simulink model "cordic_opt_fixpt16"  (R2021b)
settings: Solver=VariableStepAuto  StartTime=0.0  StopTime=116  RelTol=1e-3
undefined symbols (not defined in the file): S, vsva2197, xcvc1902
libraries: hdlBasic x7, hdlDSPIP x1, vmcUtilities x1
settings Model: Creator=shu_abe  LastModifiedBy=shu_abe

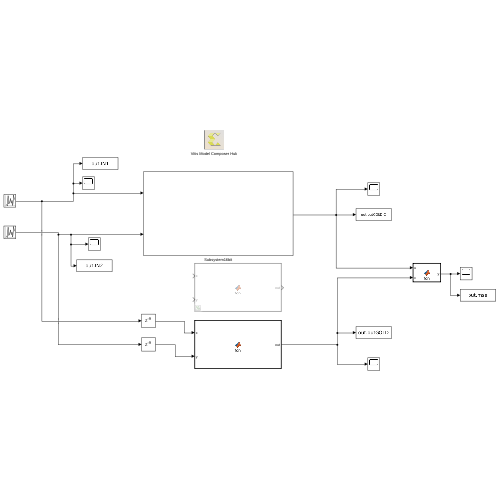
[thumbnail: Simulink's stored preview of the top-level diagram]
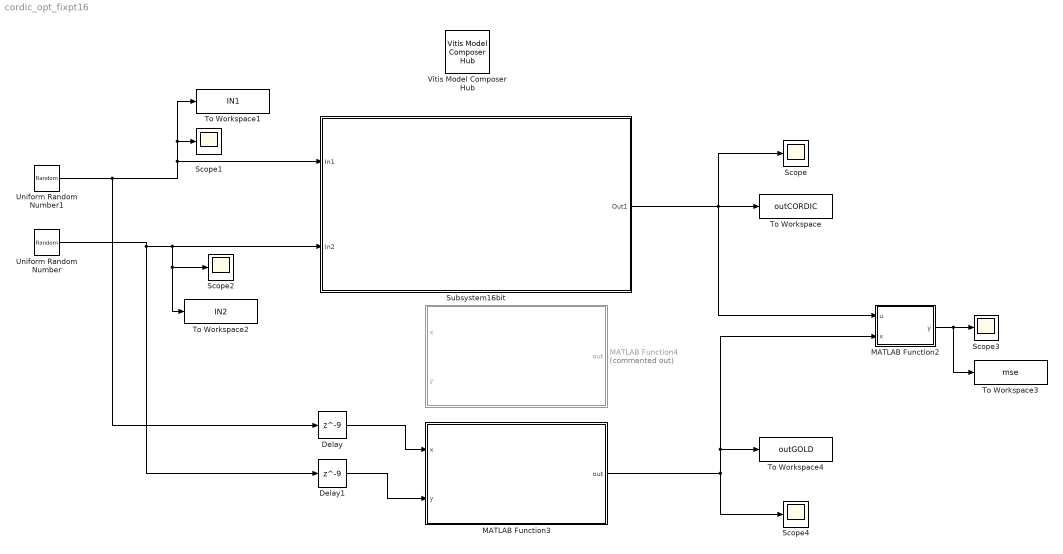
== system cordic_opt_fixpt16 ==
  Delay : Delay  DelayLength=9
  Delay1 : Delay  DelayLength=9
  MATLAB Function2 : MATLAB Function  TreatAsAtomicUnit=on
  MATLAB Function3 : MATLAB Function  TreatAsAtomicUnit=on
  MATLAB Function4 : MATLAB Function  Commented=on  TreatAsAtomicUnit=on
  Scope{,1..4} (5 alike) : Scope
  Subsystem16bit : Subsystem
      mask Display: %%%%
  To Workspace : ToWorkspace  VariableName=outCORDIC  SaveFormat=Structure With Time  SampleTime=-1
  To Workspace1 : ToWorkspace  VariableName=IN1  SaveFormat=Structure With Time  SampleTime=-1
  To Workspace2 : ToWorkspace  VariableName=IN2  SaveFormat=Structure With Time  SampleTime=-1
  To Workspace3 : ToWorkspace  VariableName=mse  SaveFormat=Structure With Time  SampleTime=-1
  To Workspace4 : ToWorkspace  VariableName=outGOLD  SaveFormat=Structure With Time  SampleTime=-1
  Uniform Random Number : UniformRandomNumber  Minimum=-0.7  Maximum=0.7  SampleTime=1
  Uniform Random Number1 : UniformRandomNumber  Minimum=-0.7  Maximum=0.7  Seed=1  SampleTime=1
  Vitis Model Composer Hub : vmcUtilities/Vitis Model Composer Hub  Tag=genX  CodeGeneration=off  SubsystemName=<enter or select subsystem name>  TargetDirectory=./code  ExportType=HLS C++ code  IpVendor=xilinx.com  IpLibrary=hls  IpVersion=1.0  IpHWLanguage=Verilog  AieCompilerOptions={}  CreateTestbench=off  TestbenchStackSize=10  RunAieSim=off  AieSimTimeout=50000  RunAieSimProfiling=off  LaunchVitisAnalyzer=off  PlotOutput=off  RunX86Sim=off  X86SimTimeout=10  GenHwImage=off  PlatformType=Not Specified  HwSystemType=Baremetal  HwValidationTarget=hw  ProjDevice=Alveo U250 Data Center Accelerator Card (xcu250-figd2104-2L-e)  ProjDevicePart=xcvc1902-vsva2197-2MP-e-S  SamplePeriod=-1  ClockFrequency=200  DataPathParallelism=1  xilinxfamily=virtexuplus  part=xcu250  speed=-2L-e  package=figd2104  directory=./cordic_optsim16  testbench=on  incr_netlist=off  synthesis_tool=Vivado  clock_wrapper=Clock Enables  dbl_ovrd=According to Block Masks  dcm_input_clock_period=10  sysclk_period=50  simulink_period=1  eval_field=0
  wires:
  Uniform Random Number/1 -> Subsystem16bit/2(In2), To Workspace2/1, Scope2/1, Delay1/1
  Uniform Random Number1/1 -> Subsystem16bit/1(In1), To Workspace1/1, Scope1/1, Delay/1
  Delay1/1 -> MATLAB Function3/2(y)
  Delay/1 -> MATLAB Function3/1(x)
  MATLAB Function3/1(out) -> Scope4/1, To Workspace4/1, MATLAB Function2/2(x)
  Subsystem16bit/1(Out1) -> Scope/1, MATLAB Function2/1(u), To Workspace/1
  MATLAB Function2/1(y) -> To Workspace3/1, Scope3/1

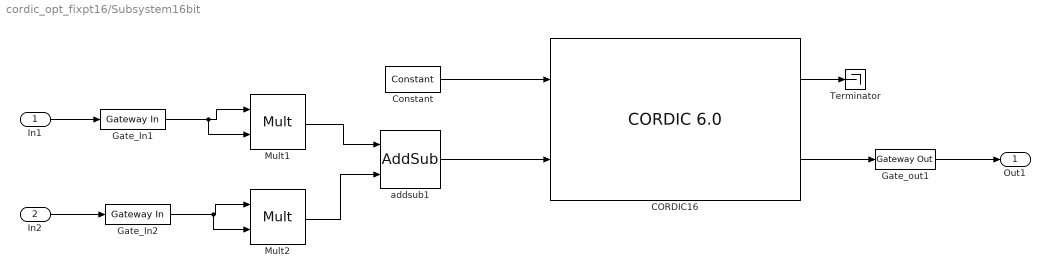
== system cordic_opt_fixpt16/Subsystem16bit ==
  In1 : Inport
  In2 : Inport  Port=2
  CORDIC16 : hdlDSPIP/CORDIC 6.0   functional_selection=Square_Root  architectural_configuration=Parallel  pipelining_mode=Optimal  data_format=UnsignedFraction  phase_format=Radians  input_width=16  output_width=16  round_mode=Round_Pos_Neg_Inf  iterations=0  precision=0  compensation_scaling=No_Scale_Compensation  coarse_rotation=off  aclken=off  aresetn=off  out_tready=off  cartesian_has_tuser=off  cartesian_has_tlast=off  cartesian_tuser_width=1  phase_has_tuser=off  phase_has_tlast=off  phase_tuser_width=1  out_tlast_behv=Null  flow_control=NonBlocking  optimize_goal=Resources  trim_axipin_name=on  simulation_type=hybrid_sim  simulation_model=sysgen:cordic_v6_0  data_path_portlist={'s_axis_cartesian_tdata_imag', 's_axis_cartesian_tdata_real', 's_axis_phase_tdata_phase', 'm_axis_dout_tdata_imag', 'm_axis_dout_tdata_real', 'm_axis_dout_tdata_phase','m_axis_dout_tdata'}  ip_name=CORDIC  ip_version=6.0  dsptool_ready=true  ipcore_usecache=true  ipcore_useipmodelcache=true  wrapper_available=true  port_translation_map={ 'aclken' => 'en', 'aresetn' => 'rst' }  XmcBlockStatus=1  maskContainerNames=group15  block_type=cordic_v6_0  block_config=sysgen:rodinimport_config  block_width=800
  Constant : hdlBasic/Constant  const=1  gui_display_data_type=Boolean  arith_type=Boolean  n_bits=16  bin_pt=14  preci_type=Single  exp_width=8  frac_width=24  explicit_period=on  period=1  XmcBlockStatus=1  maskContainerNames=tabcontainer1  block_type=constant  block_config=sysgen:Constant_config
  Gate_In1 : hdlBasic/Gateway In  gui_display_data_type=Fixed-point  arith_type=Signed (2's comp)  n_bits=16  bin_pt=14  preci_type=Single  exp_width=8  frac_width=24  rows=1  columns=1  quantization="Round  (unbiased: +/- Inf)"  overflow=Saturate  period=1  UseAsADC=off  ADCChannel='1'  interface=None  automatic_assignment=on  address_offset=hex2dec('00')  intf_name=''  intf_description=''  default_value=0  timing_constraint=None  locs_specified=off  LOCs={}  io_standard={}  inherit_from_input=off  hdl_port=on  XmcBlockStatus=1  maskContainerNames=group4  block_type=gatewayin  block_config=sysgen:gateway_in_config  block_width_w=590  block_height_w=620  block_width=640  block_height=850
  Gate_In2 : hdlBasic/Gateway In  gui_display_data_type=Fixed-point  arith_type=Signed (2's comp)  n_bits=16  bin_pt=14  preci_type=Single  exp_width=8  frac_width=24  rows=1  columns=1  quantization="Round  (unbiased: +/- Inf)"  overflow=Saturate  period=1  UseAsADC=off  ADCChannel='1'  interface=None  automatic_assignment=on  address_offset=hex2dec('00')  intf_name=''  intf_description=''  default_value=0  timing_constraint=None  locs_specified=off  LOCs={}  io_standard={}  inherit_from_input=off  hdl_port=on  XmcBlockStatus=1  maskContainerNames=group4  block_type=gatewayin  block_config=sysgen:gateway_in_config  block_width_w=590  block_height_w=620  block_width=640  block_height=850
  Gate_out1 : hdlBasic/Gateway Out  inherit_from_input=off  hdl_port=on  rows=1  columns=1  UseAsDAC=off  DACChannel='1'  interface=None  automatic_assignment=on  address_offset=hex2dec('00')  intf_name=''  intf_description=''  timing_constraint=None  locs_specified=off  LOCs={}  io_standard={}  XmcBlockStatus=1  maskContainerNames=group4  block_type=gatewayout  block_config=sysgen:gateway_out_config  block_width_w=590  block_height_w=620  block_width=620  block_height=750
  Mult1 : hdlBasic/Mult  precision=Full  arith_type="Signed  (2's comp)"  n_bits=16  bin_pt=14  quantization=Truncate  overflow=Wrap  en=off  latency=0  use_behavioral_HDL=off  opt=Area  use_embedded=off  optimum_pipeline=off  pipeline=on  use_rpm=on  placement_style=Triangular  XmcBlockStatus=1  maskContainerNames=group1  block_type=mult  block_config=sysgen:Mult_config
  Mult2 : hdlBasic/Mult  precision=Full  arith_type="Signed  (2's comp)"  n_bits=16  bin_pt=14  quantization=Truncate  overflow=Wrap  en=off  latency=0  use_behavioral_HDL=off  opt=Area  use_embedded=off  optimum_pipeline=off  pipeline=on  use_rpm=on  placement_style=Triangular  XmcBlockStatus=1  maskContainerNames=group1  block_type=mult  block_config=sysgen:Mult_config
  Terminator : Terminator
  addsub1 : hdlBasic/AddSub  mode=Addition  use_carryin=off  use_carryout=off  en=off  latency=0  precision=User Defined  arith_type=Unsigned  n_bits=16  bin_pt=15  quantization="Round  (unbiased: +/- Inf)"  overflow=Saturate  use_behavioral_HDL=off  hw_selection=Fabric  pipelined=on  XmcBlockStatus=1  maskContainerNames=tabcontainer1  block_type=addsub  block_config=sysgen:Addsub_config
  Out1 : Outport
  wires:
  CORDIC16/1 -> Terminator/1
  Gate_out1/1 -> Out1/1
  In2/1 -> Gate_In2/1
  In1/1 -> Gate_In1/1
  Gate_In2/1 -> Mult2/2, Mult2/1
  Constant/1 -> CORDIC16/1
  Mult2/1 -> addsub1/2
  Mult1/1 -> addsub1/1
  addsub1/1 -> CORDIC16/2
  Gate_In1/1 -> Mult1/2, Mult1/1
  CORDIC16/2 -> Gate_out1/1

== matlab function cordic_opt_fixpt16/MATLAB Function2 ==
  data: u input; y output; x input
function y = fcn(u,x)

y = immse(u,x);

== matlab function cordic_opt_fixpt16/MATLAB Function4 ==
  data: x input; out output; y input
function out = fcn(x,y)
tmp1 = x.^2 + y.^2;
out = cordicsqrt(tmp1);

== matlab function cordic_opt_fixpt16/MATLAB Function3 ==
  data: x input; out output; y input
function out = fcn(x,y)
out = sqrt(x.^2 + y.^2);
